simulink model "newobserversimulink_twoarea_eventtrigger"  (R2017a)
settings: Solver=ode45  StartTime=0.0  StopTime=10  RelTol=1e-3  EnableMultiTasking=on
values from neighbouring files (symbols this model uses):
  Ab = vertcat(horzcat(An,Dn),horzcat(zeros(2,9),zeros(2,2)))    [twoareaobsersimulink.m]
  An = [0 (2*pi*T1) 0 0 0 -(2*pi*T1) 0 0 0;-Kp1/Tp1 -1/Tp1 Kp1/Tp1 0 0 0 0 0 0;0 0 -1/Tch1 0 1/Tch1 0 0 0 0 ... (first row only)    [twoareaobsersimulink.m]
  Bb = vertcat(Bn,zeros(2,2))    [twoareaobsersimulink.m]
  Bn = [0 0;0 0;0 0;0 0;1/Tg1 0;0 0;0 0;0 0;0 1/Tg2]    [twoareaobsersimulink.m]
  Cb = horzcat(Cn,zeros(5,2))    [twoareaobsersimulink.m]
  Cn = [1 0 0 0 0 0 0 0 0;0 1 0 0 0 0 0 0 0;0 0 1 0 0 0 0 0 0;0 0 0 0 0 1 0 0 0;0 0 0 0 0 0 1 0 0]    [twoareaobsersimulink.m]
  Dn = [0 0;-Kp1/Tp1 0;0 0;0 0;0 0;0 -Kp2/Tp2;0 0;0 0;0 0]    [twoareaobsersimulink.m]
  h = 0.01    [twoareaobsersimulink.m]
  L = K1'    [twoareaobsersimulink.m]
libraries: powerlib x1
settings Model: Creator=Aradhnapatel  LastModifiedBy=Aradhna
settings DataIOCC: LimitDataPoints=on  SaveFormat=Array
settings OptimizationCC: LifeSpan=inf
settings DebuggingCC: UnderspecifiedInitializationDetection=Classic  MergeDetectMultiDrivingBlocksExec=none  SolverPrmCheckMsg=warning  StateNameClashWarn=warning  SFUnexpectedBacktrackingDiag=warning  SFNoUnconditionalDefaultTransitionDiag=warning  SFExecutionAtInitializationDiag=none
settings HardwareCC: ProdBitPerPointer=32  ProdBitPerSizeT=32  ProdBitPerPtrDiffT=32  ProdLargestAtomicFloat=None  ProdIntDivRoundTo=Undefined  ProdEndianess=Unspecified  ProdWordSize=32  ProdHWDeviceType=32-bit Generic
settings ModelReferenceCC: PropagateSignalLabelsOutOfModel=off
settings RTWCC: GenCodeOnly=on
settings GRTTargetCC: TargetLangStandard=C89/C90 (ANSI)  GeneratePreprocessorConditionals=Disable all
settings ConfigComp: CovMetricSettings=dw  CovHtmlReporting=on  CovSaveCumulativeToWorkspaceVar=on  CovSaveSingleToWorkspaceVar=on  CovExternalEMLEnable=off

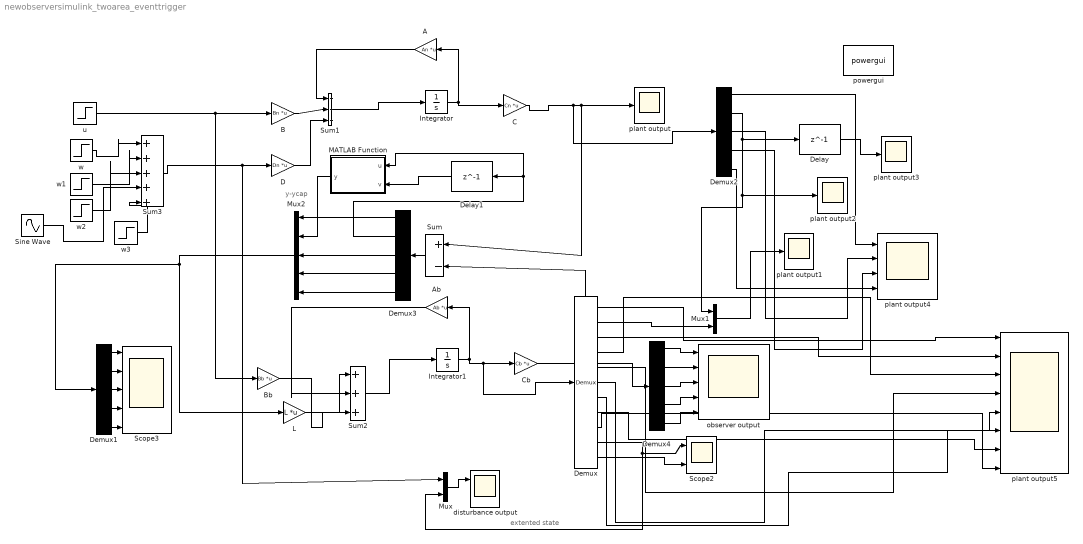
== system newobserversimulink_twoarea_eventtrigger ==
  note: extented state
  note: y-ycap
  A : Gain  Gain=An  Multiplication=Matrix(K*u)  SampleTime=h
  Ab : Gain  Gain=Ab  Multiplication=Matrix(K*u)  SampleTime=h
  B : Gain  Gain=Bn  Multiplication=Matrix(K*u)  SampleTime=h
  Bb : Gain  Gain=Bb  Multiplication=Matrix(K*u)  SampleTime=h
  C : Gain  Gain=Cn  Multiplication=Matrix(K*u)  SampleTime=h
  Cb : Gain  Gain=Cb  Multiplication=Matrix(K*u)  SampleTime=h
  D : Gain  Gain=Dn  Multiplication=Matrix(K*u)  SampleTime=h
  Delay : Delay  DelayLength=1  InitialCondition=0  InputProcessing=Columns as channels (frame based)
  Delay1 : Delay  DelayLength=1  InitialCondition=0  InputProcessing=Columns as channels (frame based)
  Demux : Demux  Outputs=11
  Demux{1..4} (4 alike) : Demux  Outputs=5
  Integrator : Integrator
  Integrator1 : Integrator  InitialCondition=[0.001;0.01;0.001;.001;.001;.01;.002;.0001;.001;.002;.001]  IgnoreLimit=on
  L : Gain  Gain=L  Multiplication=Matrix(K*u)  SampleTime=h
  MATLAB Function : MATLAB Function  TreatAsAtomicUnit=on
  Mux : Mux  Inputs=2
  Mux1 : Mux  Inputs=2
  Mux2 : Mux  Inputs=5
  Scope2 : Scope  NumInputPorts=2
  Scope3 : Scope  NumInputPorts=5
  Sine Wave : Sin  Amplitude=0  Frequency=0.5  SampleTime=0
  Sum : Sum  Inputs=|+-
  Sum1 : Sum  Inputs=|+++
  Sum2 : Sum  Inputs=|+++
  Sum3 : Sum  Inputs=|+++++
  disturbance output : Scope  NumInputPorts=2
  observer output : Scope  NumInputPorts=5
  plant output{,1..3} (4 alike) : Scope
  plant output4 : Scope  NumInputPorts=4
  plant output5 : Scope  NumInputPorts=8
  powergui : powerlib/powergui  Priority=1  SimulationMode=Discrete  SampleTime=h  frequency=60  Iterations=50  frequencyindice=60  Pbase=100e6  ErrMax=1e-4  UnitsV=kV  UnitsW=MW  buscounter=0  FunctionMessages=off  echomessages=off  EnableUseOfTLC=off  CurrentSourceSwitches=off  DisableSnubberDevices=off  DisableRonSwitches=off  DisableVfSwitches=off  DisplayEquations=off  SolverType=Tustin  Interpol=off  ExternalGateDelay=off  methode=off  Ts=0  x0status=blocks  SPID=on  SwTol=0  HookPort=off  RestoreLinks=warning  ResistiveCurrentMeasurement=off  Frange=[0:2:500]  Ylog=off  Xlog=on  ShowGrid=off  save=off  variable=ZData  structure=0  ZoomFFT=off  StartTime=0.0  cycles=1  DisplayStyle=1  fundamental=60  FreqAxis=off  MaxFrequency=1000  frequencyindicesteady=1  RmsSteady=1  display=off
  u : Step  Time=0  After=[0.00000;0.00000]  SampleTime=h  VectorParams1D=off  ZeroCross=off
  w : Step  Time=3  After=[1;1]  SampleTime=h
  w1 : Step  Time=8  After=[1;1]  SampleTime=h
  w2 : Step  Time=5  After=[1;1]  SampleTime=h
  w3 : Step  After=[1;1]  SampleTime=h
  wires:
  Integrator/1 -> C/1, A/1
  A/1 -> Sum1/1
  Sum1/1 -> Integrator/1
  B/1 -> Sum1/2
  D/1 -> Sum1/3
  Sum3/1 -> Mux/1, D/1
  Integrator1/1 -> Demux/1, Cb/1, Ab/1
  Sum2/1 -> Integrator1/1
  Demux/10 -> Mux/2, Scope2/1
  Demux/11 -> Scope2/2
  Mux/1 -> disturbance output/1
  u/1 -> Bb/1, B/1
  Demux1/1 -> Scope3/1
  Demux1/2 -> Scope3/2
  Demux1/3 -> Scope3/3
  Demux1/4 -> Scope3/4
  Demux1/5 -> Scope3/5
  w/1 -> Sum3/1
  Demux/2 -> Mux1/2
  Mux1/1 -> plant output1/1
  Demux2/2 -> plant output2/1, Mux1/1, Delay/1
  Cb/1 -> Sum/2, Demux4/1
  C/1 -> Sum/1, plant output/1, Demux2/1
  Sum/1 -> Demux3/1
  Demux3/1 -> Mux2/1
  Demux3/3 -> Mux2/3
  Demux3/4 -> Mux2/4
  Demux3/5 -> Mux2/5
  L/1 -> Sum2/1
  Bb/1 -> Sum2/3
  Ab/1 -> Sum2/2
  Demux4/1 -> observer output/1
  Demux4/2 -> observer output/2
  Demux4/3 -> observer output/3
  Demux4/4 -> observer output/4
  Demux4/5 -> observer output/5
  w1/1 -> Sum3/2
  w2/1 -> Sum3/3
  w3/1 -> Sum3/5
  Mux2/1 -> L/1, Demux1/1
  Delay/1 -> plant output3/1
  Delay1/1 -> MATLAB Function/2(v)
  Demux3/2 -> Delay1/1, MATLAB Function/1(u)
  MATLAB Function/1(y) -> Mux2/2
  Sine Wave/1 -> Sum3/4
  Demux2/1 -> plant output4/1
  Demux2/3 -> plant output4/2
  Demux2/4 -> plant output4/3
  Demux2/5 -> plant output4/4
  Demux/1 -> plant output5/1
  Demux/3 -> plant output5/2
  Demux/4 -> plant output5/3
  Demux/5 -> plant output5/4
  Demux/6 -> plant output5/5
  Demux/7 -> plant output5/6
  Demux/8 -> plant output5/7
  Demux/9 -> plant output5/8

== matlab function newobserversimulink_twoarea_eventtrigger/MATLAB Function ==
  data: u input; y output; v input
function y = fcn(u,v)
%#codegen

if abs(u)>0.0001
y = u;
else
y=u
end
